simulink model "dimensions_equivalent"  (R2021b)
settings: Solver=VariableStepAuto  StartTime=0.0  StopTime=10.0  RelTol=1e-3
undefined symbols (not defined in the file): DiscIntNeverNeededParam, magnitude, Newton, Raphson
libraries: simulink x80, slpidlib x2
(part 3 of 3)

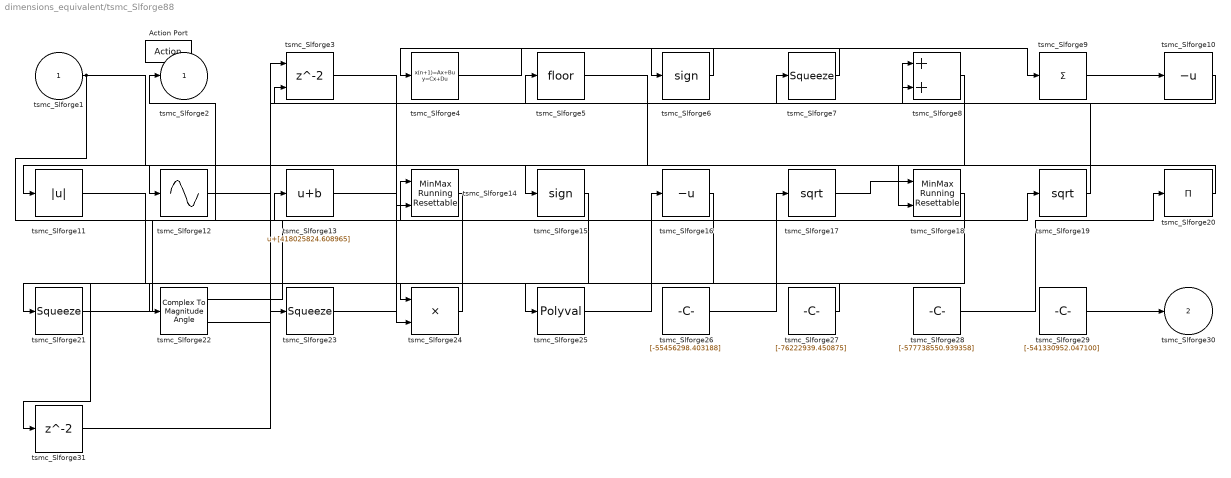
== system dimensions_equivalent/tsmc_Slforge88 ==
  tsmc_Slforge1 : Inport
  Action Port : ActionPort  ActionPortLabel=if { }
  tsmc_Slforge10 : UnaryMinus
  tsmc_Slforge11 : Abs
  tsmc_Slforge12 : Sin  TimeSource=Use external signal  SampleTime=0
  tsmc_Slforge13 : Bias  Bias=[418025824.608965]
  tsmc_Slforge14 : simulink/Math Operations/MinMax Running Resettable  Function=min  vinit=0.0
  tsmc_Slforge15 : Signum
  tsmc_Slforge16 : UnaryMinus
  tsmc_Slforge17 : Sqrt  SaturateOnIntegerOverflow=on
  tsmc_Slforge18 : simulink/Math Operations/MinMax Running Resettable  Function=min  vinit=0.0
  tsmc_Slforge19 : Sqrt  SaturateOnIntegerOverflow=on
  tsmc_Slforge20 : Product  Inputs=*
  tsmc_Slforge21 : Squeeze
  tsmc_Slforge22 : ComplexToMagnitudeAngle
  tsmc_Slforge23 : Squeeze
  tsmc_Slforge24 : Product
  tsmc_Slforge25 : Polyval  Coefs=[ +2.081618890e-019, -1.441693666e-014, +4.719686976e-010, -8.536869453e-006, +1.621573104e-001, -8.087801117e+001 ]
  tsmc_Slforge26 : Constant  Value=[-55456298.403188]  SampleTime=1
  tsmc_Slforge27 : Constant  Value=[-76222939.450875]  SampleTime=1
  tsmc_Slforge28 : Constant  Value=[-577738550.939358]  SampleTime=1
  tsmc_Slforge29 : Constant  Value=[-541330952.047100]  SampleTime=1
  tsmc_Slforge3 : Delay  ShowEnablePort=on
      settings: InputPortMap=u0,e6
  tsmc_Slforge31 : Delay
  tsmc_Slforge4 : DiscreteStateSpace  SampleTime=-1
  tsmc_Slforge5 : Rounding
  tsmc_Slforge6 : Signum
  tsmc_Slforge7 : Squeeze
  tsmc_Slforge8 : Sum
  tsmc_Slforge9 : Sum  Inputs=+
  tsmc_Slforge2 : Outport  VectorParamsAs1DForOutWhenUnconnected=off
  tsmc_Slforge30 : Outport  Port=2  VectorParamsAs1DForOutWhenUnconnected=off
  wires:
  tsmc_Slforge20/1 -> tsmc_Slforge11/1
  tsmc_Slforge1/1 -> tsmc_Slforge19/1, tsmc_Slforge15/1
  tsmc_Slforge6/1 -> tsmc_Slforge4/1
  tsmc_Slforge27/1 -> tsmc_Slforge25/1
  tsmc_Slforge25/1 -> tsmc_Slforge16/1
  tsmc_Slforge21/1 -> tsmc_Slforge13/1
  tsmc_Slforge10/1 -> tsmc_Slforge5/1
  tsmc_Slforge12/1 -> tsmc_Slforge23/1
  tsmc_Slforge22/1 -> tsmc_Slforge14/1
  tsmc_Slforge8/1 -> tsmc_Slforge12/1
  tsmc_Slforge3/1 -> tsmc_Slforge14/2
  tsmc_Slforge26/1 -> tsmc_Slforge17/1
  tsmc_Slforge24/1 -> tsmc_Slforge2/1
  tsmc_Slforge16/1 -> tsmc_Slforge22/1
  tsmc_Slforge11/1 -> tsmc_Slforge24/1
  tsmc_Slforge7/1 -> tsmc_Slforge6/1
  tsmc_Slforge23/1 -> tsmc_Slforge7/1
  tsmc_Slforge18/1 -> tsmc_Slforge24/2
  tsmc_Slforge28/1 -> tsmc_Slforge20/1
  tsmc_Slforge9/1 -> tsmc_Slforge10/1
  tsmc_Slforge15/1 -> tsmc_Slforge21/1
  tsmc_Slforge4/1 -> tsmc_Slforge9/1
  tsmc_Slforge29/1 -> tsmc_Slforge30/1
  tsmc_Slforge19/1 -> tsmc_Slforge3/2
  tsmc_Slforge13/1 -> tsmc_Slforge8/1
  tsmc_Slforge17/1 -> tsmc_Slforge18/1
  tsmc_Slforge5/1 -> tsmc_Slforge18/2
  tsmc_Slforge22/2 -> tsmc_Slforge8/2
  tsmc_Slforge14/1 -> tsmc_Slforge31/1
  tsmc_Slforge31/1 -> tsmc_Slforge3/1

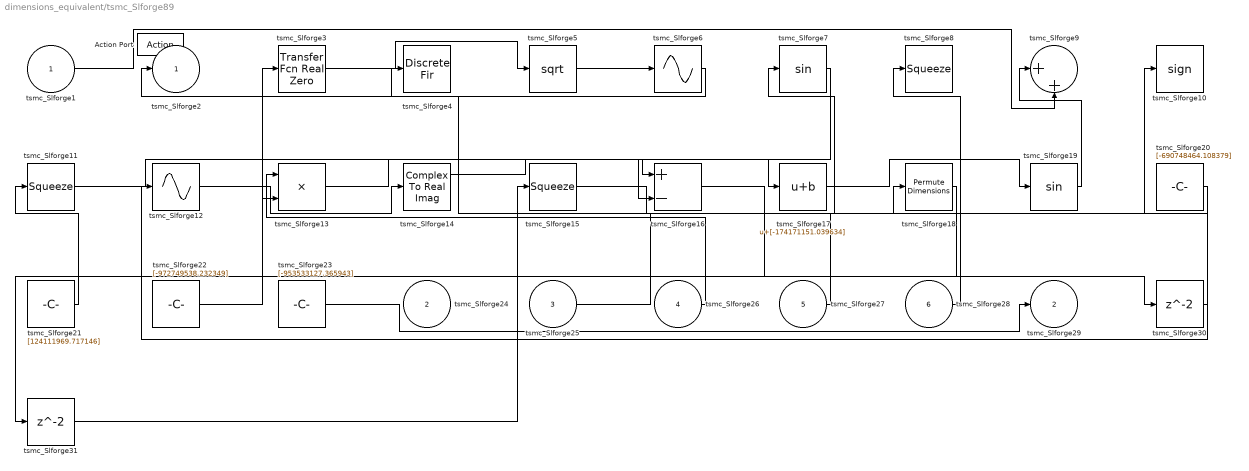
== system dimensions_equivalent/tsmc_Slforge89 ==
  tsmc_Slforge1 : Inport
  tsmc_Slforge24 : Inport  Port=2
  tsmc_Slforge25 : Inport  Port=3
  tsmc_Slforge26 : Inport  Port=4
  tsmc_Slforge27 : Inport  Port=5
  tsmc_Slforge28 : Inport  Port=6
  Action Port : ActionPort  ActionPortLabel=else { }
  tsmc_Slforge10 : Signum
  tsmc_Slforge11 : Squeeze
  tsmc_Slforge12 : Sin  TimeSource=Use external signal  SampleTime=0
  tsmc_Slforge13 : Product  Inputs=**
  tsmc_Slforge14 : ComplexToRealImag
  tsmc_Slforge15 : Squeeze
  tsmc_Slforge16 : Sum  Inputs=+-
  tsmc_Slforge17 : Bias  Bias=[-174171151.039634]
  tsmc_Slforge18 : PermuteDimensions
  tsmc_Slforge19 : Trigonometry
  tsmc_Slforge20 : Constant  Value=[-690748464.108379]  SampleTime=1
  tsmc_Slforge21 : Constant  Value=[124111969.717146]  SampleTime=1
  tsmc_Slforge22 : Constant  Value=[-972749538.232349]  SampleTime=1
  tsmc_Slforge23 : Constant  Value=[-953533127.365943]  SampleTime=1
  tsmc_Slforge3 : simulink/Discrete/Transfer Fcn Real Zero  ZeroZ=0.75  ICPrevInput=0.0  DoSatur=off
      settings: SourceProductBaseCode=SL
  tsmc_Slforge30 : Delay
  tsmc_Slforge31 : Delay
  tsmc_Slforge4 : DiscreteFir
  tsmc_Slforge5 : Sqrt  SaturateOnIntegerOverflow=on
  tsmc_Slforge6 : Sin  TimeSource=Use external signal  SampleTime=0
  tsmc_Slforge7 : Trigonometry
  tsmc_Slforge8 : Squeeze
  tsmc_Slforge9 : Sum  Inputs=|++
  tsmc_Slforge2 : Outport  VectorParamsAs1DForOutWhenUnconnected=off
  tsmc_Slforge29 : Outport  Port=2  VectorParamsAs1DForOutWhenUnconnected=off
  wires:
  tsmc_Slforge11/1 -> tsmc_Slforge17/1
  tsmc_Slforge5/1 -> tsmc_Slforge6/1
  tsmc_Slforge15/1 -> tsmc_Slforge18/1
  tsmc_Slforge28/1 -> tsmc_Slforge8/1
  tsmc_Slforge17/1 -> tsmc_Slforge19/1
  tsmc_Slforge21/1 -> tsmc_Slforge11/1
  tsmc_Slforge23/1 -> tsmc_Slforge29/1
  tsmc_Slforge6/1 -> tsmc_Slforge2/1
  tsmc_Slforge26/1 -> tsmc_Slforge13/1
  tsmc_Slforge19/1 -> tsmc_Slforge9/1
  tsmc_Slforge3/1 -> tsmc_Slforge5/1
  tsmc_Slforge12/1 -> tsmc_Slforge14/1
  tsmc_Slforge27/1 -> tsmc_Slforge4/1
  tsmc_Slforge25/1 -> tsmc_Slforge10/1
  tsmc_Slforge20/1 -> tsmc_Slforge12/1
  tsmc_Slforge13/1 -> tsmc_Slforge16/1
  tsmc_Slforge1/1 -> tsmc_Slforge9/2
  tsmc_Slforge22/1 -> tsmc_Slforge3/1
  tsmc_Slforge14/1 -> tsmc_Slforge16/2
  tsmc_Slforge7/1 -> tsmc_Slforge13/2
  tsmc_Slforge16/1 -> tsmc_Slforge30/1
  tsmc_Slforge30/1 -> tsmc_Slforge7/1
  tsmc_Slforge18/1 -> tsmc_Slforge31/1
  tsmc_Slforge31/1 -> tsmc_Slforge15/1

== system dimensions_equivalent/tsmc_Slforge90 ==
  tsmc_Slforge1 : Inport
  tsmc_Slforge23 : Inport  Port=2
  tsmc_Slforge24 : Inport  Port=3
  tsmc_Slforge25 : Inport  Port=4
  tsmc_Slforge26 : Inport  Port=5
  Action Port : ActionPort  ActionPortLabel=if { }
  tsmc_Slforge10 : Product  Inputs=*
  tsmc_Slforge11 : Rounding
  tsmc_Slforge12 : DotProduct  InputSameDT=on  OutDataTypeStr=Inherit: Inherit via internal rule
  tsmc_Slforge13 : Sum  Inputs=|++
  tsmc_Slforge14 : Squeeze
  tsmc_Slforge15 : Reshape
  tsmc_Slforge16 : Math  Operator=log  SignedPower=on  SaturateOnIntegerOverflow=on
  tsmc_Slforge17 : Trigonometry
  tsmc_Slforge18 : Sum  Inputs=+
  tsmc_Slforge19 : MinMax  Inputs=3
  tsmc_Slforge20 : Bias  Bias=[159828129.616630]
  tsmc_Slforge21 : MinMax  Function=max  Inputs=3
  tsmc_Slforge22 : Constant  Value=[-157254162.791757]  SampleTime=1
  tsmc_Slforge3 : simulink/Discrete/Transfer Fcn Lead or Lag  PoleZ=0.95  ZeroZ=0.75  ICPrevOutput=0.0  ICPrevInput=0.0  DoSatur=off
      settings: SourceProductBaseCode=SL
  tsmc_Slforge4 : DiscreteFilter
  tsmc_Slforge5 : Delay
  tsmc_Slforge6 : simulink/Continuous/PID Controller  Controller=PID  TimeDomain=Discrete-time  SampleTime=-1  IntegratorMethod=Forward Euler  FilterMethod=Forward Euler  Form=Parallel  UseFilter=on  ControllerParametersSource=internal  P=1  I=1  D=0  N=100  InitialConditionSource=internal  InitialConditionForIntegrator=0  InitialConditionForFilter=0  ExternalReset=none  LimitOutput=off  UpperSaturationLimit=inf  LowerSaturationLimit=-inf  LinearizeAsGain=off  AntiWindupMode=none  Kb=1  TrackingMode=off  Kt=1  PParamMin=[]  PParamMax=[]  IParamMin=[]  IParamMax=[]  DParamMin=[]  DParamMax=[]  NParamMin=[]  NParamMax=[]  KbParamMin=[]  KbParamMax=[]  KtParamMin=[]  KtParamMax=[]  POutMin=[]  POutMax=[]  IOutMin=[]  IOutMax=[]  DOutMin=[]  DOutMax=[]  NOutMin=[]  NOutMax=[]  KbOutMin=[]  KbOutMax=[]  KtOutMin=[]  KtOutMax=[]  IntegratorOutMin=[]  IntegratorOutMax=[]  FilterOutMin=[]  FilterOutMax=[]  SumOutMin=[]  SumOutMax=[]  SumI1OutMin=[]  SumI1OutMax=[]  SumI2OutMin=[]  SumI2OutMax=[]  SumI3OutMin=[]  SumI3OutMax=[]  SumDOutMin=[]  SumDOutMax=[]  SaturationOutMin=[]  SaturationOutMax=[]  IntegratorContinuousStateAttributes=''  IntegratorStateMustResolveToSignalObject=off  IntegratorRTWStateStorageClass=Auto  FilterContinuousStateAttributes=''  FilterStateMustResolveToSignalObject=off  FilterRTWStateStorageClass=Auto  DifferentiatorICPrevScaledInput=0  DifferentiatorOutMin=[]  DifferentiatorOutMax=[]  FilterDiffOutCoefMin=[]  FilterDiffOutCoefMax=[]  SumDenOutMin=[]  SumDenOutMax=[]  SumNumOutMin=[]  SumNumOutMax=[]  ReciprocalOutMin=[]  ReciprocalOutMax=[]  DivideOutMin=[]  DivideOutMax=[]  TunerSelectOption=Transfer Function Based (PID Tuner App)
  tsmc_Slforge7 : DotProduct  InputSameDT=on  OutDataTypeStr=Inherit: Inherit via internal rule
  tsmc_Slforge8 : Product
  tsmc_Slforge9 : ComplexToMagnitudeAngle
  tsmc_Slforge2 : Outport  VectorParamsAs1DForOutWhenUnconnected=off
  tsmc_Slforge27 : Outport  Port=2  VectorParamsAs1DForOutWhenUnconnected=off
  wires:
  tsmc_Slforge6/1 -> tsmc_Slforge13/1
  tsmc_Slforge22/1 -> tsmc_Slforge6/1
  tsmc_Slforge14/1 -> tsmc_Slforge27/1
  tsmc_Slforge19/1 -> tsmc_Slforge12/1
  tsmc_Slforge15/1 -> tsmc_Slforge16/1
  tsmc_Slforge7/1 -> tsmc_Slforge13/2
  tsmc_Slforge12/1 -> tsmc_Slforge11/1
  tsmc_Slforge20/1 -> tsmc_Slforge8/1
  tsmc_Slforge17/1 -> tsmc_Slforge15/1, tsmc_Slforge19/3
  tsmc_Slforge23/1 -> tsmc_Slforge18/1
  tsmc_Slforge18/1 -> tsmc_Slforge12/2
  tsmc_Slforge10/1 -> tsmc_Slforge8/2
  tsmc_Slforge13/1 -> tsmc_Slforge4/1
  tsmc_Slforge8/1 -> tsmc_Slforge2/1
  tsmc_Slforge11/1 -> tsmc_Slforge20/1
  tsmc_Slforge9/1 -> tsmc_Slforge7/1
  tsmc_Slforge9/2 -> tsmc_Slforge21/1
  tsmc_Slforge5/1 -> tsmc_Slforge9/1, tsmc_Slforge17/1
  tsmc_Slforge25/1 -> tsmc_Slforge14/1
  tsmc_Slforge24/1 -> tsmc_Slforge21/2, tsmc_Slforge19/2
  tsmc_Slforge4/1 -> tsmc_Slforge21/3
  tsmc_Slforge3/1 -> tsmc_Slforge10/1
  tsmc_Slforge1/1 -> tsmc_Slforge3/1
  tsmc_Slforge26/1 -> tsmc_Slforge5/1
  tsmc_Slforge16/1 -> tsmc_Slforge7/2
  tsmc_Slforge21/1 -> tsmc_Slforge19/1

== system dimensions_equivalent/tsmc_Slforge91 ==
  tsmc_Slforge1 : Inport
  tsmc_Slforge22 : Inport  Port=2
  tsmc_Slforge23 : Inport  Port=3
  tsmc_Slforge24 : Inport  Port=4
  Action Port : ActionPort  ActionPortLabel=else { }
  tsmc_Slforge10 : Gain  Gain=[-850790414.799938]
  tsmc_Slforge11 : Product
  tsmc_Slforge12 : Abs
  tsmc_Slforge13 : Trigonometry
  tsmc_Slforge14 : Squeeze
  tsmc_Slforge15 : Polyval  Coefs=[ +2.081618890e-019, -1.441693666e-014, +4.719686976e-010, -8.536869453e-006, +1.621573104e-001, -8.087801117e+001 ]
  tsmc_Slforge16 : Reshape
  tsmc_Slforge17 : Bias  Bias=[386124671.003913]
  tsmc_Slforge18 : Gain  Gain=[-965621728.411404]
  tsmc_Slforge19 : MinMax  Function=max
  tsmc_Slforge20 : Constant  Value=[-234717465.980855]  SampleTime=1
  tsmc_Slforge21 : Constant  Value=[-994967967.742177]  SampleTime=1
  tsmc_Slforge27 : Delay
  tsmc_Slforge28 : Delay
  tsmc_Slforge3 : Delay
  tsmc_Slforge4 : DiscreteFilter
  tsmc_Slforge5 : DotProduct  InputSameDT=on  OutDataTypeStr=Inherit: Inherit via internal rule
  tsmc_Slforge6 : Product  Inputs=**
  tsmc_Slforge7 : Signum
  tsmc_Slforge8 : Signum
  tsmc_Slforge9 : ComplexToMagnitudeAngle
  tsmc_Slforge2 : Outport  VectorParamsAs1DForOutWhenUnconnected=off
  tsmc_Slforge25 : Outport  Port=2  VectorParamsAs1DForOutWhenUnconnected=off
  tsmc_Slforge26 : Outport  Port=3  VectorParamsAs1DForOutWhenUnconnected=off
  wires:
  tsmc_Slforge10/1 -> tsmc_Slforge13/1
  tsmc_Slforge5/1 -> tsmc_Slforge25/1
  tsmc_Slforge13/1 -> tsmc_Slforge19/1
  tsmc_Slforge4/1 -> tsmc_Slforge12/1
  tsmc_Slforge7/1 -> tsmc_Slforge5/1
  tsmc_Slforge1/1 -> tsmc_Slforge15/1
  tsmc_Slforge15/1 -> tsmc_Slforge8/1
  tsmc_Slforge3/1 -> tsmc_Slforge5/2
  tsmc_Slforge9/1 -> tsmc_Slforge14/1
  tsmc_Slforge6/1 -> tsmc_Slforge18/1
  tsmc_Slforge12/1 -> tsmc_Slforge2/1
  tsmc_Slforge11/1 -> tsmc_Slforge16/1
  tsmc_Slforge24/1 -> tsmc_Slforge3/1
  tsmc_Slforge22/1 -> tsmc_Slforge6/1
  tsmc_Slforge9/2 -> tsmc_Slforge26/1
  tsmc_Slforge20/1 -> tsmc_Slforge11/1
  tsmc_Slforge23/1 -> tsmc_Slforge4/1
  tsmc_Slforge14/1 -> tsmc_Slforge11/2
  tsmc_Slforge21/1 -> tsmc_Slforge17/1
  tsmc_Slforge8/1 -> tsmc_Slforge7/1
  tsmc_Slforge17/1 -> tsmc_Slforge9/1
  tsmc_Slforge18/1 -> tsmc_Slforge27/1
  tsmc_Slforge27/1 -> tsmc_Slforge6/2
  tsmc_Slforge19/1 -> tsmc_Slforge28/1
  tsmc_Slforge28/1 -> tsmc_Slforge10/1

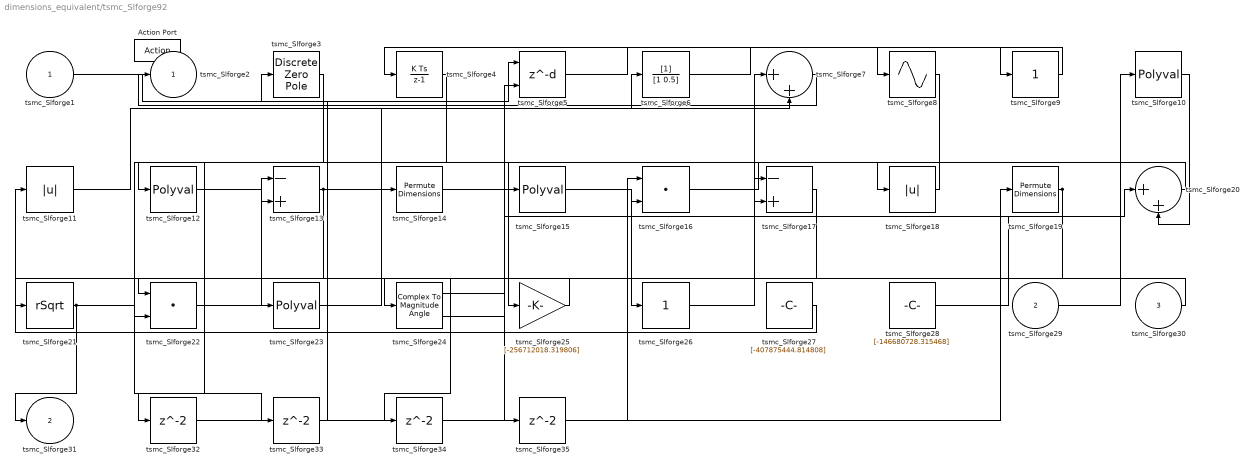
== system dimensions_equivalent/tsmc_Slforge92 ==
  tsmc_Slforge1 : Inport
  tsmc_Slforge29 : Inport  Port=2
  tsmc_Slforge30 : Inport  Port=3
  Action Port : ActionPort  ActionPortLabel=if { }
  tsmc_Slforge{10,12,15,23} (4 alike) : Polyval  Coefs=[ +2.081618890e-019, -1.441693666e-014, +4.719686976e-010, -8.536869453e-006, +1.621573104e-001, -8.087801117e+001 ]
  tsmc_Slforge11 : Abs
  tsmc_Slforge13 : Sum  Inputs=-+
  tsmc_Slforge14 : PermuteDimensions
  tsmc_Slforge16 : DotProduct  InputSameDT=on  OutDataTypeStr=Inherit: Inherit via internal rule
  tsmc_Slforge17 : Sum  Inputs=-+
  tsmc_Slforge18 : Abs
  tsmc_Slforge19 : PermuteDimensions
  tsmc_Slforge20 : Sum  Inputs=|++
  tsmc_Slforge21 : Sqrt  Operator=rSqrt  AlgorithmType=Newton-Raphson  SaturateOnIntegerOverflow=on
  tsmc_Slforge22 : DotProduct  InputSameDT=on  OutDataTypeStr=Inherit: Inherit via internal rule
  tsmc_Slforge24 : ComplexToMagnitudeAngle
  tsmc_Slforge25 : Gain  Gain=[-256712018.319806]
  tsmc_Slforge26 : simulink/Math Operations/Slider Gain  gain=1  low=0  high=2
  tsmc_Slforge27 : Constant  Value=[-407875444.814808]  SampleTime=1
  tsmc_Slforge28 : Constant  Value=[-146680728.315468]  SampleTime=1
  tsmc_Slforge3 : DiscreteZeroPole  Poles=[0 0.5]  Gain=1  SampleTime=-1
  tsmc_Slforge{32..35} (4 alike) : Delay
  tsmc_Slforge4 : DiscreteIntegrator  SampleTime=-1  ICPrevOutput=DiscIntNeverNeededParam  ICPrevScaledInput=DiscIntNeverNeededParam
  tsmc_Slforge5 : Delay  DelayLengthSource=Input port
      settings: InputPortMap=u0,p1
  tsmc_Slforge6 : DiscreteFilter
  tsmc_Slforge7 : Sum  Inputs=|++
  tsmc_Slforge8 : Sin  TimeSource=Use external signal  SampleTime=0
  tsmc_Slforge9 : simulink/Math Operations/Slider Gain  gain=1  low=0  high=2
  tsmc_Slforge2 : Outport  VectorParamsAs1DForOutWhenUnconnected=off
  tsmc_Slforge31 : Outport  Port=2  VectorParamsAs1DForOutWhenUnconnected=off
  wires:
  tsmc_Slforge9/1 -> tsmc_Slforge4/1
  tsmc_Slforge20/1 -> tsmc_Slforge12/1
  tsmc_Slforge30/1 -> tsmc_Slforge22/1
  tsmc_Slforge14/1 -> tsmc_Slforge25/1
  tsmc_Slforge22/1 -> tsmc_Slforge13/1
  tsmc_Slforge25/1 -> tsmc_Slforge23/1
  tsmc_Slforge1/1 -> tsmc_Slforge5/1
  tsmc_Slforge26/1 -> tsmc_Slforge7/1
  tsmc_Slforge27/1 -> tsmc_Slforge11/1
  tsmc_Slforge6/1 -> tsmc_Slforge8/1
  tsmc_Slforge11/1 -> tsmc_Slforge6/1
  tsmc_Slforge5/1 -> tsmc_Slforge9/1
  tsmc_Slforge16/1 -> tsmc_Slforge18/1
  tsmc_Slforge3/1 -> tsmc_Slforge22/2
  tsmc_Slforge13/1 -> tsmc_Slforge14/1, tsmc_Slforge21/1
  tsmc_Slforge19/1 -> tsmc_Slforge24/1, tsmc_Slforge16/2
  tsmc_Slforge7/1 -> tsmc_Slforge2/1
  tsmc_Slforge12/1 -> tsmc_Slforge13/2
  tsmc_Slforge28/1 -> tsmc_Slforge20/1
  tsmc_Slforge15/1 -> tsmc_Slforge26/1
  tsmc_Slforge10/1 -> tsmc_Slforge20/2
  tsmc_Slforge8/1 -> tsmc_Slforge15/1
  tsmc_Slforge18/1 -> tsmc_Slforge17/1
  tsmc_Slforge29/1 -> tsmc_Slforge10/1
  tsmc_Slforge23/1 -> tsmc_Slforge7/2
  tsmc_Slforge24/2 -> tsmc_Slforge17/2
  tsmc_Slforge21/1 -> tsmc_Slforge31/1, tsmc_Slforge33/1
  tsmc_Slforge4/1 -> tsmc_Slforge32/1
  tsmc_Slforge32/1 -> tsmc_Slforge5/2
  tsmc_Slforge33/1 -> tsmc_Slforge3/1
  tsmc_Slforge17/1 -> tsmc_Slforge34/1
  tsmc_Slforge34/1 -> tsmc_Slforge16/1
  tsmc_Slforge24/1 -> tsmc_Slforge35/1
  tsmc_Slforge35/1 -> tsmc_Slforge19/1

== system dimensions_equivalent/tsmc_Slforge93 ==
  tsmc_Slforge1 : Inport
  tsmc_Slforge21 : Inport  Port=2
  tsmc_Slforge22 : Inport  Port=3
  tsmc_Slforge23 : Inport  Port=4
  Action Port : ActionPort  ActionPortLabel=else { }
  tsmc_Slforge10 : Sum  Inputs=|++
  tsmc_Slforge11 : Bias  Bias=[-390575493.818071]
  tsmc_Slforge12 : simulink/Math Operations/MinMax Running Resettable  Function=min  vinit=0.0
  tsmc_Slforge13 : ComplexToRealImag
  tsmc_Slforge14 : Abs
  tsmc_Slforge15 : Squeeze
  tsmc_Slforge16 : Squeeze
  tsmc_Slforge17 : Polyval  Coefs=[ +2.081618890e-019, -1.441693666e-014, +4.719686976e-010, -8.536869453e-006, +1.621573104e-001, -8.087801117e+001 ]
  tsmc_Slforge18 : Polyval  Coefs=[ +2.081618890e-019, -1.441693666e-014, +4.719686976e-010, -8.536869453e-006, +1.621573104e-001, -8.087801117e+001 ]
  tsmc_Slforge19 : Constant  Value=[296436115.168826]  SampleTime=1
  tsmc_Slforge20 : Constant  Value=[801294350.649234]  SampleTime=1
  tsmc_Slforge24 : Delay
  tsmc_Slforge25 : Delay
  tsmc_Slforge3 : Delay  DelayLengthSource=Input port
      settings: InputPortMap=u0,p1
  tsmc_Slforge4 : DiscreteFir
  tsmc_Slforge5 : Delay  DelayLengthSource=Input port
      settings: InputPortMap=u0,p1
  tsmc_Slforge6 : Trigonometry
  tsmc_Slforge7 : MinMax  Inputs=2
  tsmc_Slforge8 : Trigonometry
  tsmc_Slforge9 : Rounding
  tsmc_Slforge2 : Outport  VectorParamsAs1DForOutWhenUnconnected=off
  wires:
  tsmc_Slforge16/1 -> tsmc_Slforge9/1
  tsmc_Slforge11/1 -> tsmc_Slforge17/1
  tsmc_Slforge12/1 -> tsmc_Slforge2/1
  tsmc_Slforge1/1 -> tsmc_Slforge11/1
  tsmc_Slforge7/1 -> tsmc_Slforge5/1
  tsmc_Slforge13/1 -> tsmc_Slforge14/1
  tsmc_Slforge22/1 -> tsmc_Slforge3/1
  tsmc_Slforge21/1 -> tsmc_Slforge4/1
  tsmc_Slforge14/1 -> tsmc_Slforge16/1
  tsmc_Slforge4/1 -> tsmc_Slforge7/1
  tsmc_Slforge13/2 -> tsmc_Slforge7/2
  tsmc_Slforge3/1 -> tsmc_Slforge12/1
  tsmc_Slforge10/1 -> tsmc_Slforge18/1
  tsmc_Slforge19/1 -> tsmc_Slforge3/2
  tsmc_Slforge15/1 -> tsmc_Slforge13/1
  tsmc_Slforge23/1 -> tsmc_Slforge5/2
  tsmc_Slforge17/1 -> tsmc_Slforge12/2
  tsmc_Slforge20/1 -> tsmc_Slforge10/2
  tsmc_Slforge5/1 -> tsmc_Slforge8/1
  tsmc_Slforge6/1 -> tsmc_Slforge15/1
  tsmc_Slforge9/1 -> tsmc_Slforge24/1
  tsmc_Slforge24/1 -> tsmc_Slforge6/1
  tsmc_Slforge18/1 -> tsmc_Slforge25/1
  tsmc_Slforge25/1 -> tsmc_Slforge10/1

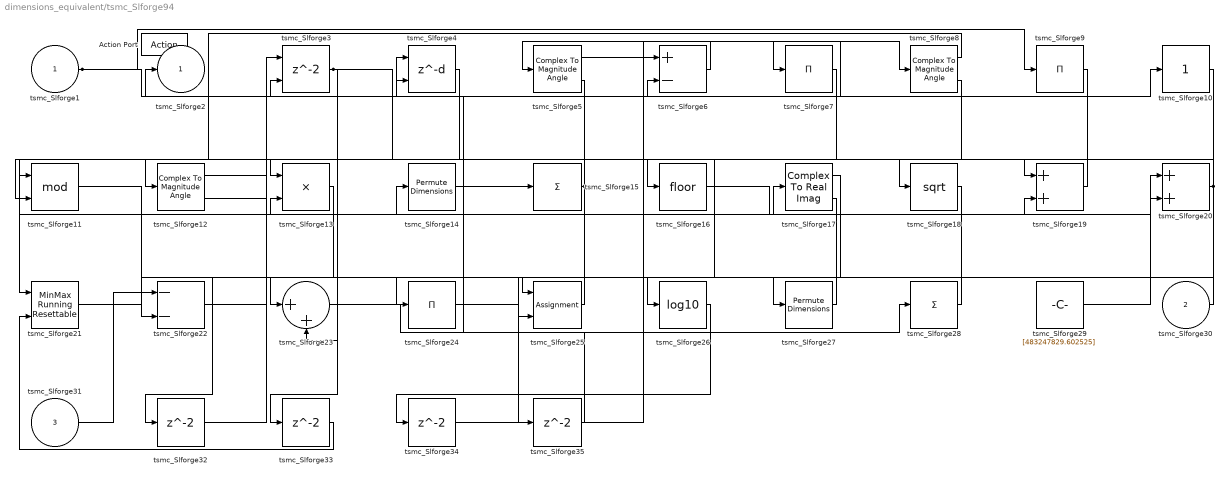
== system dimensions_equivalent/tsmc_Slforge94 ==
  tsmc_Slforge1 : Inport
  tsmc_Slforge30 : Inport  Port=2
  tsmc_Slforge31 : Inport  Port=3
  Action Port : ActionPort  ActionPortLabel=if { }
  tsmc_Slforge10 : simulink/Math Operations/Slider Gain  gain=1  low=0  high=2
  tsmc_Slforge11 : Math  Operator=mod  SignedPower=on  SaturateOnIntegerOverflow=on
  tsmc_Slforge12 : ComplexToMagnitudeAngle
  tsmc_Slforge13 : Product  Inputs=**
  tsmc_Slforge14 : PermuteDimensions
  tsmc_Slforge15 : Sum  Inputs=+
  tsmc_Slforge16 : Rounding
  tsmc_Slforge17 : ComplexToRealImag
  tsmc_Slforge18 : Sqrt  SaturateOnIntegerOverflow=on
  tsmc_Slforge19 : Sum
  tsmc_Slforge20 : Sum
  tsmc_Slforge21 : simulink/Math Operations/MinMax Running Resettable  Function=min  vinit=0.0
  tsmc_Slforge22 : Sum  Inputs=--
  tsmc_Slforge23 : Sum  Inputs=|++
  tsmc_Slforge24 : Product  Inputs=*
  tsmc_Slforge25 : Assignment  DiagnosticForDimensions=Warning  IndexOptions=Index vector (dialog)  Indices=1  OutputSizes=1
  tsmc_Slforge26 : Math  Operator=log10  SignedPower=on  SaturateOnIntegerOverflow=on
  tsmc_Slforge27 : PermuteDimensions
  tsmc_Slforge28 : Sum  Inputs=+
  tsmc_Slforge29 : Constant  Value=[483247829.602525]  SampleTime=1
  tsmc_Slforge3 : Delay  ShowEnablePort=on
      settings: InputPortMap=u0,e6
  tsmc_Slforge{32..35} (4 alike) : Delay
  tsmc_Slforge4 : Delay  DelayLengthSource=Input port
      settings: InputPortMap=u0,p1
  tsmc_Slforge5 : ComplexToMagnitudeAngle
  tsmc_Slforge6 : Sum  Inputs=+-
  tsmc_Slforge7 : Product  Inputs=*
  tsmc_Slforge8 : ComplexToMagnitudeAngle
  tsmc_Slforge9 : Product  Inputs=*
  tsmc_Slforge2 : Outport  VectorParamsAs1DForOutWhenUnconnected=off
  wires:
  tsmc_Slforge14/1 -> tsmc_Slforge15/1
  tsmc_Slforge7/1 -> tsmc_Slforge13/1
  tsmc_Slforge31/1 -> tsmc_Slforge22/1
  tsmc_Slforge19/1 -> tsmc_Slforge7/1
  tsmc_Slforge18/1 -> tsmc_Slforge17/1
  tsmc_Slforge25/1 -> tsmc_Slforge4/1
  tsmc_Slforge1/1 -> tsmc_Slforge9/1, tsmc_Slforge10/1
  tsmc_Slforge8/1 -> tsmc_Slforge21/1
  tsmc_Slforge11/1 -> tsmc_Slforge22/2
  tsmc_Slforge10/1 -> tsmc_Slforge16/1
  tsmc_Slforge15/1 -> tsmc_Slforge4/2, tsmc_Slforge24/1
  tsmc_Slforge21/1 -> tsmc_Slforge27/1
  tsmc_Slforge27/1 -> tsmc_Slforge3/2
  tsmc_Slforge23/1 -> tsmc_Slforge28/1
  tsmc_Slforge28/1 -> tsmc_Slforge13/2
  tsmc_Slforge8/2 -> tsmc_Slforge26/1
  tsmc_Slforge3/1 -> tsmc_Slforge19/1, tsmc_Slforge33/1
  tsmc_Slforge12/1 -> tsmc_Slforge18/1
  tsmc_Slforge20/1 -> tsmc_Slforge12/1, tsmc_Slforge23/2
  tsmc_Slforge5/1 -> tsmc_Slforge8/1
  tsmc_Slforge30/1 -> tsmc_Slforge25/1
  tsmc_Slforge4/1 -> tsmc_Slforge23/1
  tsmc_Slforge22/1 -> tsmc_Slforge6/2
  tsmc_Slforge17/1 -> tsmc_Slforge25/2
  tsmc_Slforge6/1 -> tsmc_Slforge5/1
  tsmc_Slforge29/1 -> tsmc_Slforge20/1
  tsmc_Slforge16/1 -> tsmc_Slforge20/2
  tsmc_Slforge12/2 -> tsmc_Slforge19/2
  tsmc_Slforge17/2 -> tsmc_Slforge11/1
  tsmc_Slforge5/2 -> tsmc_Slforge2/1
  tsmc_Slforge9/1 -> tsmc_Slforge11/2
  tsmc_Slforge13/1 -> tsmc_Slforge32/1
  tsmc_Slforge32/1 -> tsmc_Slforge3/1
  tsmc_Slforge33/1 -> tsmc_Slforge21/2
  tsmc_Slforge26/1 -> tsmc_Slforge34/1
  tsmc_Slforge34/1 -> tsmc_Slforge6/1
  tsmc_Slforge24/1 -> tsmc_Slforge35/1
  tsmc_Slforge35/1 -> tsmc_Slforge14/1

== system dimensions_equivalent/tsmc_Slforge95 ==
  tsmc_Slforge1 : Inport
  tsmc_Slforge26 : Inport  Port=2
  tsmc_Slforge27 : Inport  Port=3
  tsmc_Slforge28 : Inport  Port=4
  Action Port : ActionPort  ActionPortLabel=else { }
  tsmc_Slforge10 : Squeeze
  tsmc_Slforge11 : Sum  Inputs=|++
  tsmc_Slforge12 : Polyval  Coefs=[ +2.081618890e-019, -1.441693666e-014, +4.719686976e-010, -8.536869453e-006, +1.621573104e-001, -8.087801117e+001 ]
  tsmc_Slforge13 : Abs
  tsmc_Slforge14 : simulink/Math Operations/Slider Gain  gain=1  low=0  high=2
  tsmc_Slforge15 : simulink/Math Operations/Slider Gain  gain=1  low=0  high=2
  tsmc_Slforge16 : ComplexToMagnitudeAngle
  tsmc_Slforge17 : Assignment  DiagnosticForDimensions=Warning  IndexOptions=Index vector (dialog)  Indices=1  OutputSizes=1
  tsmc_Slforge18 : UnaryMinus
  tsmc_Slforge19 : Assignment  DiagnosticForDimensions=Warning  IndexOptions=Index vector (dialog)  Indices=1  OutputSizes=1
  tsmc_Slforge20 : Sqrt  SaturateOnIntegerOverflow=on
  tsmc_Slforge21 : Math  Operator=10^u  SignedPower=on  SaturateOnIntegerOverflow=on
  tsmc_Slforge22 : Math  Operator=rem  SignedPower=on  SaturateOnIntegerOverflow=on
  tsmc_Slforge23 : Assignment  DiagnosticForDimensions=Warning  IndexOptions=Index vector (dialog)  Indices=1  OutputSizes=1
  tsmc_Slforge24 : Product  Inputs=**
  tsmc_Slforge25 : Gain  Gain=[-241050901.710005]
  tsmc_Slforge3 : DiscreteFilter
  tsmc_Slforge30 : Delay
  tsmc_Slforge31 : Delay
  tsmc_Slforge4 : simulink/Discrete/Transfer Fcn Lead or Lag  PoleZ=0.95  ZeroZ=0.75  ICPrevOutput=0.0  ICPrevInput=0.0  DoSatur=off
      settings: SourceProductBaseCode=SL
  tsmc_Slforge5 : Product  Inputs=**
  tsmc_Slforge6 : UnaryMinus
  tsmc_Slforge7 : Sin  TimeSource=Use external signal  SampleTime=0
  tsmc_Slforge8 : Sum  Inputs=|++
  tsmc_Slforge9 : Abs
  tsmc_Slforge2 : Outport  VectorParamsAs1DForOutWhenUnconnected=off
  tsmc_Slforge29 : Outport  Port=2  VectorParamsAs1DForOutWhenUnconnected=off
  wires:
  tsmc_Slforge3/1 -> tsmc_Slforge21/1
  tsmc_Slforge13/1 -> tsmc_Slforge10/1, tsmc_Slforge15/1
  tsmc_Slforge16/1 -> tsmc_Slforge7/1
  tsmc_Slforge1/1 -> tsmc_Slforge11/1
  tsmc_Slforge28/1 -> tsmc_Slforge20/1
  tsmc_Slforge26/1 -> tsmc_Slforge4/1
  tsmc_Slforge21/1 -> tsmc_Slforge5/1
  tsmc_Slforge8/1 -> tsmc_Slforge17/1
  tsmc_Slforge12/1 -> tsmc_Slforge24/1
  tsmc_Slforge10/1 -> tsmc_Slforge3/1
  tsmc_Slforge18/1 -> tsmc_Slforge16/1
  tsmc_Slforge7/1 -> tsmc_Slforge29/1
  tsmc_Slforge9/1 -> tsmc_Slforge23/1
  tsmc_Slforge20/1 -> tsmc_Slforge9/1, tsmc_Slforge2/1
  tsmc_Slforge23/1 -> tsmc_Slforge24/2
  tsmc_Slforge17/1 -> tsmc_Slforge14/1
  tsmc_Slforge19/1 -> tsmc_Slforge13/1
  tsmc_Slforge11/1 -> tsmc_Slforge18/1, tsmc_Slforge17/2, tsmc_Slforge19/2
  tsmc_Slforge6/1 -> tsmc_Slforge12/1
  tsmc_Slforge4/1 -> tsmc_Slforge6/1
  tsmc_Slforge24/1 -> tsmc_Slforge22/1
  tsmc_Slforge25/1 -> tsmc_Slforge23/2
  tsmc_Slforge16/2 -> tsmc_Slforge8/1
  tsmc_Slforge15/1 -> tsmc_Slforge5/2, tsmc_Slforge22/2
  tsmc_Slforge22/1 -> tsmc_Slforge8/2
  tsmc_Slforge27/1 -> tsmc_Slforge25/1
  tsmc_Slforge14/1 -> tsmc_Slforge30/1
  tsmc_Slforge30/1 -> tsmc_Slforge11/2
  tsmc_Slforge5/1 -> tsmc_Slforge31/1
  tsmc_Slforge31/1 -> tsmc_Slforge19/1

== system dimensions_equivalent/tsmc_Slforge96 ==
  tsmc_Slforge1 : Inport
  tsmc_Slforge29 : Inport  Port=2
  Action Port : ActionPort  ActionPortLabel=if { }
  tsmc_Slforge10 : Squeeze
  tsmc_Slforge11 : Polyval  Coefs=[ +2.081618890e-019, -1.441693666e-014, +4.719686976e-010, -8.536869453e-006, +1.621573104e-001, -8.087801117e+001 ]
  tsmc_Slforge12 : Product  Inputs=*
  tsmc_Slforge13 : Product  Inputs=**
  tsmc_Slforge14 : Sum  Inputs=+
  tsmc_Slforge15 : Math  Operator=conj  SignedPower=on  SaturateOnIntegerOverflow=on
  tsmc_Slforge16 : Rounding
  tsmc_Slforge17 : PermuteDimensions
  tsmc_Slforge18 : PermuteDimensions
  tsmc_Slforge19 : Abs
  tsmc_Slforge20 : Trigonometry
  tsmc_Slforge21 : Polyval  Coefs=[ +2.081618890e-019, -1.441693666e-014, +4.719686976e-010, -8.536869453e-006, +1.621573104e-001, -8.087801117e+001 ]
  tsmc_Slforge22 : UnaryMinus
  tsmc_Slforge23 : Sqrt  SaturateOnIntegerOverflow=on
  tsmc_Slforge24 : Product  Inputs=*
  tsmc_Slforge25 : Gain  Gain=[195514505.361535]
  tsmc_Slforge26 : Reshape
  tsmc_Slforge27 : Product  Inputs=*
  tsmc_Slforge28 : Constant  Value=[336232862.689419]  SampleTime=1
  tsmc_Slforge3 : simulink/Discrete/Transfer Fcn First Order  PoleZ=0.95  ICPrevOutput=0.0  DoSatur=off
  tsmc_Slforge30 : Delay
  tsmc_Slforge31 : Delay
  tsmc_Slforge4 : Product
  tsmc_Slforge5 : Sqrt  Operator=rSqrt  AlgorithmType=Newton-Raphson  SaturateOnIntegerOverflow=on
  tsmc_Slforge6 : Sum  Inputs=+
  tsmc_Slforge7 : simulink/Math Operations/MinMax Running Resettable  Function=min  vinit=0.0
  tsmc_Slforge8 : simulink/Math Operations/Slider Gain  gain=1  low=0  high=2
  tsmc_Slforge9 : Squeeze
  tsmc_Slforge2 : Outport  VectorParamsAs1DForOutWhenUnconnected=off
  wires:
  tsmc_Slforge8/1 -> tsmc_Slforge19/1
  tsmc_Slforge29/1 -> tsmc_Slforge27/1
  tsmc_Slforge25/1 -> tsmc_Slforge17/1
  tsmc_Slforge20/1 -> tsmc_Slforge11/1
  tsmc_Slforge1/1 -> tsmc_Slforge5/1
  tsmc_Slforge15/1 -> tsmc_Slforge18/1
  tsmc_Slforge7/1 -> tsmc_Slforge9/1
  tsmc_Slforge27/1 -> tsmc_Slforge24/1
  tsmc_Slforge14/1 -> tsmc_Slforge23/1
  tsmc_Slforge6/1 -> tsmc_Slforge10/1
  tsmc_Slforge13/1 -> tsmc_Slforge20/1
  tsmc_Slforge24/1 -> tsmc_Slforge3/1
  tsmc_Slforge28/1 -> tsmc_Slforge21/1
  tsmc_Slforge17/1 -> tsmc_Slforge7/1
  tsmc_Slforge22/1 -> tsmc_Slforge14/1
  tsmc_Slforge3/1 -> tsmc_Slforge13/1
  tsmc_Slforge18/1 -> tsmc_Slforge22/1, tsmc_Slforge4/2
  tsmc_Slforge10/1 -> tsmc_Slforge25/1
  tsmc_Slforge21/1 -> tsmc_Slforge16/1
  tsmc_Slforge23/1 -> tsmc_Slforge12/1
  tsmc_Slforge19/1 -> tsmc_Slforge6/1
  tsmc_Slforge12/1 -> tsmc_Slforge2/1
  tsmc_Slforge5/1 -> tsmc_Slforge8/1
  tsmc_Slforge9/1 -> tsmc_Slforge15/1
  tsmc_Slforge16/1 -> tsmc_Slforge4/1
  tsmc_Slforge4/1 -> tsmc_Slforge26/1
  tsmc_Slforge26/1 -> tsmc_Slforge30/1
  tsmc_Slforge30/1 -> tsmc_Slforge7/2
  tsmc_Slforge11/1 -> tsmc_Slforge31/1
  tsmc_Slforge31/1 -> tsmc_Slforge13/2

== system dimensions_equivalent/tsmc_Slforge97 ==
  tsmc_Slforge1 : Inport
  tsmc_Slforge25 : Inport  Port=2
  Action Port : ActionPort  ActionPortLabel=else { }
  tsmc_Slforge10 : UnaryMinus
  tsmc_Slforge11 : Math  Operator=mod  SignedPower=on  SaturateOnIntegerOverflow=on
  tsmc_Slforge{7,12,16,21} (4 alike) : Sqrt  Operator=rSqrt  AlgorithmType=Newton-Raphson  SaturateOnIntegerOverflow=on
  tsmc_Slforge13 : Product  Inputs=*
  tsmc_Slforge14 : Sum  Inputs=-+
  tsmc_Slforge15 : Squeeze
  tsmc_Slforge17 : DotProduct  InputSameDT=on  OutDataTypeStr=Inherit: Inherit via internal rule
  tsmc_Slforge18 : Reshape
  tsmc_Slforge19 : Sqrt  SaturateOnIntegerOverflow=on
  tsmc_Slforge20 : Product
  tsmc_Slforge22 : Product
  tsmc_Slforge23 : Sum  Inputs=+
  tsmc_Slforge24 : Constant  Value=[-511493439.314214]  SampleTime=1
  tsmc_Slforge{26..30} (5 alike) : Delay
  tsmc_Slforge3 : simulink/Continuous/PID Controller (2DOF)  Controller=PID  TimeDomain=Discrete-time  SampleTime=-1  IntegratorMethod=Forward Euler  FilterMethod=Forward Euler  Form=Parallel  UseFilter=on  ControllerParametersSource=internal  P=1  I=1  D=0  N=100  b=1  c=1  InitialConditionSource=internal  InitialConditionForIntegrator=0  InitialConditionForFilter=0  ExternalReset=none  LimitOutput=off  UpperSaturationLimit=inf  LowerSaturationLimit=-inf  LinearizeAsGain=off  AntiWindupMode=none  Kb=1  TrackingMode=off  Kt=1  PParamMin=[]  PParamMax=[]  IParamMin=[]  IParamMax=[]  DParamMin=[]  DParamMax=[]  NParamMin=[]  NParamMax=[]  bParamMin=[]  bParamMax=[]  cParamMin=[]  cParamMax=[]  KbParamMin=[]  KbParamMax=[]  KtParamMin=[]  KtParamMax=[]  POutMin=[]  POutMax=[]  IOutMin=[]  IOutMax=[]  DOutMin=[]  DOutMax=[]  NOutMin=[]  NOutMax=[]  bOutMin=[]  bOutMax=[]  cOutMin=[]  cOutMax=[]  KbOutMin=[]  KbOutMax=[]  KtOutMin=[]  KtOutMax=[]  IntegratorOutMin=[]  IntegratorOutMax=[]  FilterOutMin=[]  FilterOutMax=[]  SumOutMin=[]  SumOutMax=[]  Sum1OutMin=[]  Sum1OutMax=[]  Sum2OutMin=[]  Sum2OutMax=[]  Sum3OutMin=[]  Sum3OutMax=[]  SumI1OutMin=[]  SumI1OutMax=[]  SumI2OutMin=[]  SumI2OutMax=[]  SumI3OutMin=[]  SumI3OutMax=[]  SumDOutMin=[]  SumDOutMax=[]  SaturationOutMin=[]  SaturationOutMax=[]  IntegratorContinuousStateAttributes=''  IntegratorStateMustResolveToSignalObject=off  IntegratorRTWStateStorageClass=Auto  FilterContinuousStateAttributes=''  FilterStateMustResolveToSignalObject=off  FilterRTWStateStorageClass=Auto  DifferentiatorICPrevScaledInput=0  DifferentiatorOutMin=[]  DifferentiatorOutMax=[]  FilterDiffOutCoefMin=[]  FilterDiffOutCoefMax=[]  SumDenOutMin=[]  SumDenOutMax=[]  SumNumOutMin=[]  SumNumOutMax=[]  ReciprocalOutMin=[]  ReciprocalOutMax=[]  DivideOutMin=[]  DivideOutMax=[]  TunerSelectOption=Transfer Function Based (PID Tuner App)
  tsmc_Slforge4 : Math  Operator=transpose  SignedPower=on  SaturateOnIntegerOverflow=on
  tsmc_Slforge5 : Product
  tsmc_Slforge6 : Gain  Gain=[-111827001.508387]
  tsmc_Slforge8 : Product  Inputs=**
  tsmc_Slforge9 : Assignment  DiagnosticForDimensions=Warning  IndexOptions=Index vector (dialog)  Indices=1  OutputSizes=1
  tsmc_Slforge2 : Outport  VectorParamsAs1DForOutWhenUnconnected=off
  wires:
  tsmc_Slforge25/1 -> tsmc_Slforge12/1
  tsmc_Slforge17/1 -> tsmc_Slforge14/1
  tsmc_Slforge14/1 -> tsmc_Slforge10/1, tsmc_Slforge21/1
  tsmc_Slforge6/1 -> tsmc_Slforge9/1
  tsmc_Slforge15/1 -> tsmc_Slforge6/1, tsmc_Slforge17/1
  tsmc_Slforge20/1 -> tsmc_Slforge17/2, tsmc_Slforge27/1
  tsmc_Slforge11/1 -> tsmc_Slforge20/1
  tsmc_Slforge24/1 -> tsmc_Slforge2/1
  tsmc_Slforge4/1 -> tsmc_Slforge22/2, tsmc_Slforge14/2
  tsmc_Slforge22/1 -> tsmc_Slforge3/1
  tsmc_Slforge9/1 -> tsmc_Slforge18/1
  tsmc_Slforge19/1 -> tsmc_Slforge23/1
  tsmc_Slforge3/1 -> tsmc_Slforge11/2, tsmc_Slforge26/1
  tsmc_Slforge7/1 -> tsmc_Slforge4/1
  tsmc_Slforge12/1 -> tsmc_Slforge3/2
  tsmc_Slforge23/1 -> tsmc_Slforge8/2
  tsmc_Slforge5/1 -> tsmc_Slforge15/1
  tsmc_Slforge10/1 -> tsmc_Slforge16/1, tsmc_Slforge13/1
  tsmc_Slforge1/1 -> tsmc_Slforge19/1
  tsmc_Slforge8/1 -> tsmc_Slforge5/1, tsmc_Slforge11/1
  tsmc_Slforge18/1 -> tsmc_Slforge7/1
  tsmc_Slforge26/1 -> tsmc_Slforge9/2
  tsmc_Slforge27/1 -> tsmc_Slforge22/1
  tsmc_Slforge16/1 -> tsmc_Slforge28/1
  tsmc_Slforge28/1 -> tsmc_Slforge5/2
  tsmc_Slforge13/1 -> tsmc_Slforge29/1
  tsmc_Slforge29/1 -> tsmc_Slforge8/1
  tsmc_Slforge21/1 -> tsmc_Slforge30/1
  tsmc_Slforge30/1 -> tsmc_Slforge20/2

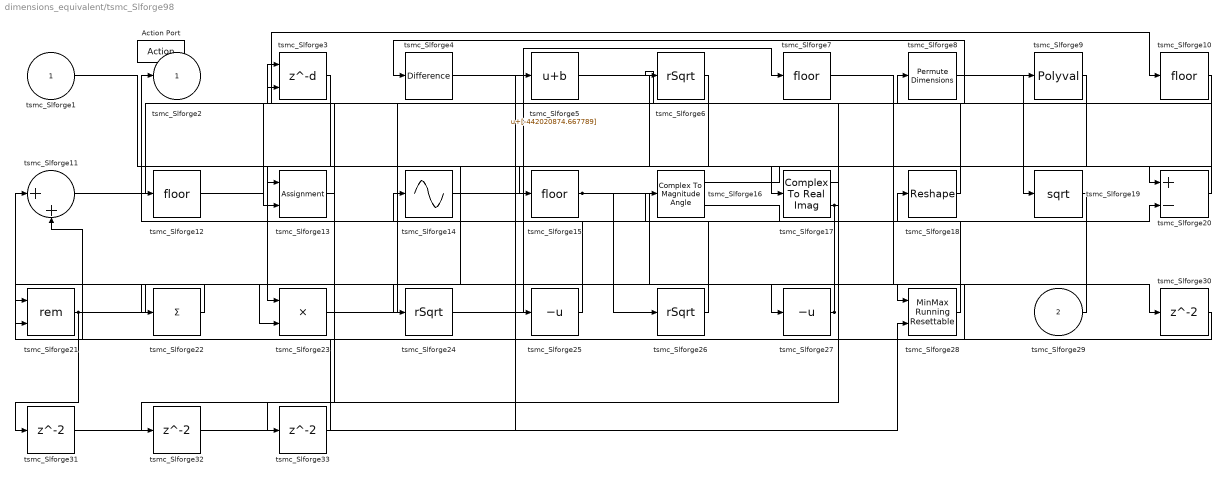
== system dimensions_equivalent/tsmc_Slforge98 ==
  tsmc_Slforge1 : Inport
  tsmc_Slforge29 : Inport  Port=2
  Action Port : ActionPort  ActionPortLabel=if { }
  tsmc_Slforge{7,10,12,15} (4 alike) : Rounding
  tsmc_Slforge11 : Sum  Inputs=|++
  tsmc_Slforge13 : Assignment  DiagnosticForDimensions=Warning  IndexOptions=Index vector (dialog)  Indices=1  OutputSizes=1
  tsmc_Slforge14 : Sin  TimeSource=Use external signal  SampleTime=0
  tsmc_Slforge16 : ComplexToMagnitudeAngle
  tsmc_Slforge17 : ComplexToRealImag
  tsmc_Slforge18 : Reshape
  tsmc_Slforge19 : Sqrt  SaturateOnIntegerOverflow=on
  tsmc_Slforge20 : Sum  Inputs=+-
  tsmc_Slforge21 : Math  Operator=rem  SignedPower=on  SaturateOnIntegerOverflow=on
  tsmc_Slforge22 : Sum  Inputs=+
  tsmc_Slforge23 : Product  Inputs=**
  tsmc_Slforge24 : Sqrt  Operator=rSqrt  AlgorithmType=Newton-Raphson  SaturateOnIntegerOverflow=on
  tsmc_Slforge25 : UnaryMinus
  tsmc_Slforge26 : Sqrt  Operator=rSqrt  AlgorithmType=Newton-Raphson  SaturateOnIntegerOverflow=on
  tsmc_Slforge27 : UnaryMinus
  tsmc_Slforge28 : simulink/Math Operations/MinMax Running Resettable  Function=min  vinit=0.0
  tsmc_Slforge3 : Delay  DelayLengthSource=Input port
      settings: InputPortMap=u0,p1
  tsmc_Slforge{30..33} (4 alike) : Delay
  tsmc_Slforge4 : simulink/Discrete/Difference  ICPrevInput=0.0  OutMin=[]  OutMax=[]  OutDataTypeStr=Inherit: Inherit via back propagation  OutDataType=fixdt(1, 16)  OutScaling=2^-10  DoSatur=off
  tsmc_Slforge5 : Bias  Bias=[-442020874.667789]
  tsmc_Slforge6 : Sqrt  Operator=rSqrt  AlgorithmType=Newton-Raphson  SaturateOnIntegerOverflow=on
  tsmc_Slforge8 : PermuteDimensions
  tsmc_Slforge9 : Polyval  Coefs=[ +2.081618890e-019, -1.441693666e-014, +4.719686976e-010, -8.536869453e-006, +1.621573104e-001, -8.087801117e+001 ]
  tsmc_Slforge2 : Outport  VectorParamsAs1DForOutWhenUnconnected=off
  wires:
  tsmc_Slforge15/1 -> tsmc_Slforge28/1, tsmc_Slforge26/1
  tsmc_Slforge5/1 -> tsmc_Slforge17/1
  tsmc_Slforge18/1 -> tsmc_Slforge6/1
  tsmc_Slforge3/1 -> tsmc_Slforge23/1
  tsmc_Slforge24/1 -> tsmc_Slforge7/1
  tsmc_Slforge19/1 -> tsmc_Slforge11/1
  tsmc_Slforge21/1 -> tsmc_Slforge23/2, tsmc_Slforge31/1
  tsmc_Slforge20/1 -> tsmc_Slforge4/1
  tsmc_Slforge11/1 -> tsmc_Slforge10/1
  tsmc_Slforge8/1 -> tsmc_Slforge19/1
  tsmc_Slforge25/1 -> tsmc_Slforge2/1
  tsmc_Slforge16/1 -> tsmc_Slforge20/1
  tsmc_Slforge29/1 -> tsmc_Slforge18/1
  tsmc_Slforge23/1 -> tsmc_Slforge9/1
  tsmc_Slforge10/1 -> tsmc_Slforge13/1
  tsmc_Slforge22/1 -> tsmc_Slforge21/1
  tsmc_Slforge14/1 -> tsmc_Slforge27/1
  tsmc_Slforge28/1 -> tsmc_Slforge14/1
  tsmc_Slforge16/2 -> tsmc_Slforge20/2
  tsmc_Slforge17/2 -> tsmc_Slforge3/1, tsmc_Slforge12/1
  tsmc_Slforge1/1 -> tsmc_Slforge15/1
  tsmc_Slforge27/1 -> tsmc_Slforge22/1, tsmc_Slforge16/1
  tsmc_Slforge4/1 -> tsmc_Slforge25/1
  tsmc_Slforge26/1 -> tsmc_Slforge3/2
  tsmc_Slforge12/1 -> tsmc_Slforge8/1
  tsmc_Slforge9/1 -> tsmc_Slforge24/1
  tsmc_Slforge6/1 -> tsmc_Slforge13/2
  tsmc_Slforge7/1 -> tsmc_Slforge30/1
  tsmc_Slforge30/1 -> tsmc_Slforge21/2
  tsmc_Slforge31/1 -> tsmc_Slforge28/2
  tsmc_Slforge17/1 -> tsmc_Slforge32/1
  tsmc_Slforge32/1 -> tsmc_Slforge5/1
  tsmc_Slforge13/1 -> tsmc_Slforge33/1
  tsmc_Slforge33/1 -> tsmc_Slforge11/2

== system dimensions_equivalent/tsmc_Slforge99 ==
  tsmc_Slforge1 : Inport
  tsmc_Slforge26 : Inport  Port=2
  tsmc_Slforge27 : Inport  Port=3
  tsmc_Slforge28 : Inport  Port=4
  Action Port : ActionPort  ActionPortLabel=else { }
  tsmc_Slforge10 : Product
  tsmc_Slforge11 : Rounding
  tsmc_Slforge12 : Sum  Inputs=+-
  tsmc_Slforge13 : Product  Inputs=**
  tsmc_Slforge14 : Sqrt  SaturateOnIntegerOverflow=on
  tsmc_Slforge15 : Sum  Inputs=|++
  tsmc_Slforge16 : Product  Inputs=**
  tsmc_Slforge17 : simulink/Math Operations/MinMax Running Resettable  Function=min  vinit=0.0
  tsmc_Slforge18 : Abs
  tsmc_Slforge19 : UnaryMinus
  tsmc_Slforge20 : Sum
  tsmc_Slforge21 : Assignment  DiagnosticForDimensions=Warning  IndexOptions=Index vector (dialog)  Indices=1  OutputSizes=1
  tsmc_Slforge22 : MinMax
  tsmc_Slforge23 : Polyval  Coefs=[ +2.081618890e-019, -1.441693666e-014, +4.719686976e-010, -8.536869453e-006, +1.621573104e-001, -8.087801117e+001 ]
  tsmc_Slforge24 : Sum  Inputs=+
  tsmc_Slforge25 : Constant  Value=[611988040.780699]  SampleTime=1
  tsmc_Slforge29 : Delay
  tsmc_Slforge3 : DiscreteZeroPole  Poles=[0 0.5]  Gain=1  SampleTime=-1
  tsmc_Slforge4 : Delay  ShowEnablePort=on
      settings: InputPortMap=u0,e6
  tsmc_Slforge5 : UnitDelay  SampleTime=-1  HasFrameUpgradeWarning=on
  tsmc_Slforge6 : Sqrt  SaturateOnIntegerOverflow=on
  tsmc_Slforge7 : Sum
  tsmc_Slforge8 : Polyval  Coefs=[ +2.081618890e-019, -1.441693666e-014, +4.719686976e-010, -8.536869453e-006, +1.621573104e-001, -8.087801117e+001 ]
  tsmc_Slforge9 : Sum  Inputs=+-
  tsmc_Slforge2 : Outport  VectorParamsAs1DForOutWhenUnconnected=off
  wires:
  tsmc_Slforge7/1 -> tsmc_Slforge5/1
  tsmc_Slforge1/1 -> tsmc_Slforge11/1
  tsmc_Slforge23/1 -> tsmc_Slforge3/1
  tsmc_Slforge13/1 -> tsmc_Slforge2/1
  tsmc_Slforge3/1 -> tsmc_Slforge22/1
  tsmc_Slforge19/1 -> tsmc_Slforge10/1, tsmc_Slforge20/2
  tsmc_Slforge27/1 -> tsmc_Slforge18/1, tsmc_Slforge13/2
  tsmc_Slforge22/1 -> tsmc_Slforge8/1
  tsmc_Slforge16/1 -> tsmc_Slforge15/1
  tsmc_Slforge28/1 -> tsmc_Slforge10/2, tsmc_Slforge16/2
  tsmc_Slforge26/1 -> tsmc_Slforge23/1
  tsmc_Slforge10/1 -> tsmc_Slforge15/2
  tsmc_Slforge18/1 -> tsmc_Slforge12/1, tsmc_Slforge9/2
  tsmc_Slforge24/1 -> tsmc_Slforge21/1
  tsmc_Slforge5/1 -> tsmc_Slforge4/1
  tsmc_Slforge6/1 -> tsmc_Slforge14/1
  tsmc_Slforge4/1 -> tsmc_Slforge6/1
  tsmc_Slforge12/1 -> tsmc_Slforge4/2
  tsmc_Slforge9/1 -> tsmc_Slforge20/1
  tsmc_Slforge25/1 -> tsmc_Slforge24/1, tsmc_Slforge21/2
  tsmc_Slforge20/1 -> tsmc_Slforge13/1
  tsmc_Slforge21/1 -> tsmc_Slforge17/1
  tsmc_Slforge11/1 -> tsmc_Slforge19/1
  tsmc_Slforge17/1 -> tsmc_Slforge9/1, tsmc_Slforge7/2
  tsmc_Slforge8/1 -> tsmc_Slforge16/1, tsmc_Slforge12/2
  tsmc_Slforge15/1 -> tsmc_Slforge17/2
  tsmc_Slforge14/1 -> tsmc_Slforge29/1
  tsmc_Slforge29/1 -> tsmc_Slforge7/1
